simulink model "kranTest"  (R2018b)
settings: Solver=VariableStepAuto  StartTime=0.0  StopTime=Tsim  FixedStep=0.005  RelTol=1e-4
model workspace: external: MATLAB File kran_DataFile.m (data not in the file)
values from neighbouring files (symbols this model uses):
  refPointsVector = [pointThree, pointOne, pointThree, pointTwo, pointThree]    [simulate_driving.m]    (also in testDriving.m)
  Ts = 50e-3    (= 0.05)    [simulation_params.m]    (also in testDriving.m = 0.1)
undefined symbols (not defined in the file or in its folder): EvaluateTrajectory, smiData, X, Y, Z
libraries: sm_lib x105, nesl_utility x32, fl_lib x27, sh_lib x9, elec_lib x2
(part 4 of 4)

== system kranTest/Crane/Crane Mechanics/hidraulicki_trans2_2/cilindar_trans2_1_RIGID ==
  ReferenceFrame : sm_lib/Frames and Transforms/Reference Frame
  Solid : sm_lib/Body Elements/Solid  InertiaType=Custom  Mass=smiData.Solid(2).mass  MassUnits=kg  CenterOfMass=smiData.Solid(2).CoM  CenterOfMassUnits=mm  MomentsOfInertia=smiData.Solid(2).MoI  MomentsOfInertiaUnits=kg*mm^2  ProductsOfInertia=smiData.Solid(2).PoI  ProductsOfInertiaUnits=kg*mm^2  BasedOnType=Density  Density=1000  DensityUnits=kg/m^3  DoExposeReferenceFrame=on  SerializedFrames=<Frames/>  GraphicType=FromGeometry  MarkerShape=Sphere  MarkerSize=10  GraphicVisPropType=SimpleVisualProperties  GraphicDiffuseColor=smiData.Solid(2).color  GraphicSpecularColor=[0.5 0.5 0.5 1.0]  GraphicAmbientColor=[0.15 0.15 0.15 1.0]  GraphicEmissiveColor=[0.0 0.0 0.0 1.0]  GraphicShininess=75  GraphicOpacity=smiData.Solid(2).opacity  GeometryShape=FromFile  RectangleSize=[1 1]  RectangleSizeUnits=m  BrickDimensions=[1 1 1]  BrickDimensionUnits=m  CylinderRadius=1  CylinderRadiusUnits=m  CylinderLength=1  CylinderLengthUnits=m  SphereRadius=1  SphereRadiusUnits=m  EllipsoidRadii=[1 1 1]  EllipsoidRadiiUnits=m  ExtrusionCrossSection=[1 1; -1 1; -1 -1; 1 -1]  ExtrusionCrossSectionUnits=m  ExtrusionLength=1  ExtrusionLengthUnits=m  PolygonNumSides=3  PolygonOuterRadius=1  PolygonOuterRadiusUnits=m  ExtGeomFileType=STEP  ExtGeomFileName=STEPfiles/cilindar_trans2_Default_sldprt.STEP  ExtGeomFileUnits=m  RevolutionCrossSection=[1 1; 1 -1; 2 -1; 2 1]  RevolutionCrossSectionUnits=m  RevolutionExtent=Full  RevolutionAngle=180  RevolutionAngleUnits=deg
  Transform : sm_lib/Frames and Transforms/Rigid Transform  TranslationMethod=Cartesian  TranslationStandardOffset=0  TranslationLengthUnit=mm  TranslationStandardAxis=+Z  TranslationCartesianOffset=smiData.RigidTransform(2).translation  TranslationROffset=0  TranslationROffsetUnits=m  TranslationZOffset=0  TranslationZOffsetUnits=m  TranslationThetaOffset=0  TranslationThetaOffsetUnits=deg  RotationMethod=ArbitraryAxis  RotationAngleUnits=rad  RotationStandardAxis=+Z  RotationAngle=smiData.RigidTransform(2).angle  RotationArbitraryAxis=smiData.RigidTransform(2).axis  FollAlignAxisA=+X  BaseAlignAxisA=+Y  FollAlignAxisB=+Y  BaseAlignAxisB=+Z  RotationSequenceAxes=FollowerAxes  RotationSequence=XYX  RotationSequenceAngles=[0 0 0]  RotationSequenceAnglesUnits=deg  RotationMatrix=[1 0 0; 0 1 0; 0 0 1]
  Transform1 : sm_lib/Frames and Transforms/Rigid Transform  TranslationMethod=Cartesian  TranslationStandardOffset=0  TranslationLengthUnit=mm  TranslationStandardAxis=+Z  TranslationCartesianOffset=smiData.RigidTransform(20).translation  TranslationROffset=0  TranslationROffsetUnits=m  TranslationZOffset=0  TranslationZOffsetUnits=m  TranslationThetaOffset=0  TranslationThetaOffsetUnits=deg  RotationMethod=ArbitraryAxis  RotationAngleUnits=rad  RotationStandardAxis=+Z  RotationAngle=smiData.RigidTransform(20).angle  RotationArbitraryAxis=smiData.RigidTransform(20).axis  FollAlignAxisA=+X  BaseAlignAxisA=+Y  FollAlignAxisB=+Y  BaseAlignAxisB=+Z  RotationSequenceAxes=FollowerAxes  RotationSequence=XYX  RotationSequenceAngles=[0 0 0]  RotationSequenceAnglesUnits=deg  RotationMatrix=[1 0 0; 0 1 0; 0 0 1]
  F2 : PMIOPort  Side=Left
  F1 : PMIOPort  Port=2  Side=Left
  F : PMIOPort  Port=3  Side=Left
  connections:
  Solid/RConn1 -- ReferenceFrame/RConn1 -- Transform/LConn1 -- Transform1/LConn1 -- F2/RConn1
  Transform/RConn1 -- F/RConn1
  Transform1/RConn1 -- F1/RConn1

== system kranTest/Crane/Crane Mechanics/hidraulicki_trans2_2/klip_trans2_1_RIGID ==
  ReferenceFrame : sm_lib/Frames and Transforms/Reference Frame
  Solid : sm_lib/Body Elements/Solid  InertiaType=Custom  Mass=smiData.Solid(3).mass  MassUnits=kg  CenterOfMass=smiData.Solid(3).CoM  CenterOfMassUnits=mm  MomentsOfInertia=smiData.Solid(3).MoI  MomentsOfInertiaUnits=kg*mm^2  ProductsOfInertia=smiData.Solid(3).PoI  ProductsOfInertiaUnits=kg*mm^2  BasedOnType=Density  Density=1000  DensityUnits=kg/m^3  DoExposeReferenceFrame=on  SerializedFrames=<Frames/>  GraphicType=FromGeometry  MarkerShape=Sphere  MarkerSize=10  GraphicVisPropType=SimpleVisualProperties  GraphicDiffuseColor=smiData.Solid(3).color  GraphicSpecularColor=[0.5 0.5 0.5 1.0]  GraphicAmbientColor=[0.15 0.15 0.15 1.0]  GraphicEmissiveColor=[0.0 0.0 0.0 1.0]  GraphicShininess=75  GraphicOpacity=smiData.Solid(3).opacity  GeometryShape=FromFile  RectangleSize=[1 1]  RectangleSizeUnits=m  BrickDimensions=[1 1 1]  BrickDimensionUnits=m  CylinderRadius=1  CylinderRadiusUnits=m  CylinderLength=1  CylinderLengthUnits=m  SphereRadius=1  SphereRadiusUnits=m  EllipsoidRadii=[1 1 1]  EllipsoidRadiiUnits=m  ExtrusionCrossSection=[1 1; -1 1; -1 -1; 1 -1]  ExtrusionCrossSectionUnits=m  ExtrusionLength=1  ExtrusionLengthUnits=m  PolygonNumSides=3  PolygonOuterRadius=1  PolygonOuterRadiusUnits=m  ExtGeomFileType=STEP  ExtGeomFileName=STEPfiles/klip_trans2_Default_sldprt.STEP  ExtGeomFileUnits=m  RevolutionCrossSection=[1 1; 1 -1; 2 -1; 2 1]  RevolutionCrossSectionUnits=m  RevolutionExtent=Full  RevolutionAngle=180  RevolutionAngleUnits=deg
  Transform : sm_lib/Frames and Transforms/Rigid Transform  TranslationMethod=Cartesian  TranslationStandardOffset=0  TranslationLengthUnit=mm  TranslationStandardAxis=+Z  TranslationCartesianOffset=smiData.RigidTransform(1).translation  TranslationROffset=0  TranslationROffsetUnits=m  TranslationZOffset=0  TranslationZOffsetUnits=m  TranslationThetaOffset=0  TranslationThetaOffsetUnits=deg  RotationMethod=ArbitraryAxis  RotationAngleUnits=rad  RotationStandardAxis=+Z  RotationAngle=smiData.RigidTransform(1).angle  RotationArbitraryAxis=smiData.RigidTransform(1).axis  FollAlignAxisA=+X  BaseAlignAxisA=+Y  FollAlignAxisB=+Y  BaseAlignAxisB=+Z  RotationSequenceAxes=FollowerAxes  RotationSequence=XYX  RotationSequenceAngles=[0 0 0]  RotationSequenceAnglesUnits=deg  RotationMatrix=[1 0 0; 0 1 0; 0 0 1]
  Transform1 : sm_lib/Frames and Transforms/Rigid Transform  TranslationMethod=Cartesian  TranslationStandardOffset=0  TranslationLengthUnit=mm  TranslationStandardAxis=+Z  TranslationCartesianOffset=smiData.RigidTransform(10).translation  TranslationROffset=0  TranslationROffsetUnits=m  TranslationZOffset=0  TranslationZOffsetUnits=m  TranslationThetaOffset=0  TranslationThetaOffsetUnits=deg  RotationMethod=ArbitraryAxis  RotationAngleUnits=rad  RotationStandardAxis=+Z  RotationAngle=smiData.RigidTransform(10).angle  RotationArbitraryAxis=smiData.RigidTransform(10).axis  FollAlignAxisA=+X  BaseAlignAxisA=+Y  FollAlignAxisB=+Y  BaseAlignAxisB=+Z  RotationSequenceAxes=FollowerAxes  RotationSequence=XYX  RotationSequenceAngles=[0 0 0]  RotationSequenceAnglesUnits=deg  RotationMatrix=[1 0 0; 0 1 0; 0 0 1]
  F1 : PMIOPort  Side=Left
  F : PMIOPort  Port=2  Side=Right
  connections:
  Solid/RConn1 -- ReferenceFrame/RConn1 -- Transform/LConn1 -- Transform1/LConn1
  Transform/RConn1 -- F/RConn1
  Transform1/RConn1 -- F1/RConn1

== matlab function kranTest/ControllerTrans1/RegulatorTrans1 ==
  data: t input; coordNum input; y output; pos input; vel input; load_pos input; load_vel input; top_pos input; top_vel input
function y = trans1(t, coordNum, pos, vel, load_pos, load_vel, top_pos, top_vel)

% Hardcode references
actuatorRefOne = [0, 0.7, 3.4, 3.4, 6150];
actuatorRefTwo = [-135, 0.415, 3.4, 3.4, 4300];
actuatorRefThree = [-90, 0.8, 0, 0, 2000];
actuatorRefVector = [actuatorRefThree; actuatorRefOne,; actuatorRefThree; actuatorRefTwo; actuatorRefThree];

baseRef = actuatorRefVector(coordNum, 1);
rotRef = actuatorRefVector(coordNum, 2);
trans1Ref = actuatorRefVector(coordNum, 3);
trans2Ref = actuatorRefVector(coordNum, 4);
pulleyRef = actuatorRefVector(coordNum, 5);

% Measurement extraction
rotPos = pos(1);
trans1Pos = pos(2);
trans2Pos = pos(3);
baseAngle = pos(4);
pulleyAngle = pos(5);

rotVel = vel(1);
tran1Vel = vel(2);
trans2Vel = vel(3);
baseVel = vel(4);
pulleyVel = vel(5);

deltaRot = rotRef - rotPos;
if (abs(deltaRot) > 0.005)
    y = 0;
else
    deltaTrans1 = trans1Ref - trans1Pos;
    if(abs(deltaTrans1) <= 0.005)
        y = 0;
    else
        y = 0.005*sign(deltaTrans1);
    end
end

end

== matlab function kranTest/ControllerRot/RegulatorRot ==
  data: t input; coordNum input; y output; pos input; vel input; load_pos input; load_vel input; top_pos input; top_vel input
function y = rot(t, coordNum, pos, vel, load_pos, load_vel, top_pos, top_vel)

% Hardcode references
actuatorRefOne = [0, 0.7, 3.4, 3.4, 6150];
actuatorRefTwo = [-135, 0.415, 3.4, 3.4, 4300];
actuatorRefThree = [-90, 0.8, 0, 0, 2000];
actuatorRefVector = [actuatorRefThree; actuatorRefOne,; actuatorRefThree; actuatorRefTwo; actuatorRefThree];

baseRef = actuatorRefVector(coordNum, 1);
rotRef = actuatorRefVector(coordNum, 2);
trans1Ref = actuatorRefVector(coordNum, 3);
trans2Ref = actuatorRefVector(coordNum, 4);
pulleyRef = actuatorRefVector(coordNum, 5);

% Measurement extraction
rotPos = pos(1);
trans1Pos = pos(2);
trans2Pos = pos(3);
baseAngle = pos(4);
pulleyAngle = pos(5);

rotVel = vel(1);
tran1Vel = vel(2);
trans2Vel = vel(3);
baseVel = vel(4);
pulleyVel = vel(5);

delta = rotRef - rotPos;
if(abs(delta) <= 0.005)
    y = 0;
else
    y = 0.003*sign(delta);
end

end

== matlab function kranTest/ControllerTrans2/RegulatorTrans2 ==
  data: t input; coordNum input; y output; pos input; vel input; load_pos input; load_vel input; top_pos input; top_vel input
function y = trans2(t, coordNum, pos, vel, load_pos, load_vel, top_pos, top_vel)

% Hardcode references
actuatorRefOne = [0, 0.7, 3.4, 3.4, 6150];
actuatorRefTwo = [-135, 0.415, 3.4, 3.4, 4300];
actuatorRefThree = [-90, 0.8, 0, 0, 2000];
actuatorRefVector = [actuatorRefThree; actuatorRefOne,; actuatorRefThree; actuatorRefTwo; actuatorRefThree];

baseRef = actuatorRefVector(coordNum, 1);
rotRef = actuatorRefVector(coordNum, 2);
trans1Ref = actuatorRefVector(coordNum, 3);
trans2Ref = actuatorRefVector(coordNum, 4);
pulleyRef = actuatorRefVector(coordNum, 5);

% Measurement extraction
rotPos = pos(1);
trans1Pos = pos(2);
trans2Pos = pos(3);
baseAngle = pos(4);
pulleyAngle = pos(5);

rotVel = vel(1);
tran1Vel = vel(2);
trans2Vel = vel(3);
baseVel = vel(4);
pulleyVel = vel(5);

deltaRot = rotRef - rotPos;
deltaTrans1 = trans1Ref - trans1Pos;
if (abs(deltaRot) > 0.005 || abs(deltaTrans1) > 0.005)
    y = 0;
else
    deltaTrans2 = trans2Ref - trans2Pos;
    if(abs(deltaTrans2) <= 0.005)
        y = 0;
    else
        y = 0.005*sign(deltaTrans2);
    end
end

end

== matlab function kranTest/ControllerBase/RegulatorBase ==
  data: t input; coordNum input; y output; pos input; vel input; load_pos input; load_vel input; top_pos input; top_vel input
function y = base(t, coordNum, pos, vel, load_pos, load_vel, top_pos, top_vel)

% Hardcode references
actuatorRefOne = [0, 0.7, 3.4, 3.4, 6150];
actuatorRefTwo = [-135, 0.415, 3.4, 3.4, 4300];
actuatorRefThree = [-90, 0.8, 0, 0, 2000];
actuatorRefVector = [actuatorRefThree; actuatorRefOne,; actuatorRefThree; actuatorRefTwo; actuatorRefThree];

baseRef = actuatorRefVector(coordNum, 1);
rotRef = actuatorRefVector(coordNum, 2);
trans1Ref = actuatorRefVector(coordNum, 3);
trans2Ref = actuatorRefVector(coordNum, 4);
pulleyRef = actuatorRefVector(coordNum, 5);

% Measurement extraction
rotPos = pos(1);
trans1Pos = pos(2);
trans2Pos = pos(3);
baseAngle = pos(4);
pulleyAngle = pos(5);

rotVel = vel(1);
tran1Vel = vel(2);
trans2Vel = vel(3);
baseVel = vel(4);
pulleyVel = vel(5);

deltaTrans2 = trans2Ref - trans2Pos;
delta = baseRef/180*pi - baseAngle;
y = 150*delta;

end

== matlab function kranTest/ControllerPulley/RegulatorPulley ==
  data: t input; coordNum input; y output; pos input; vel input; load_pos input; load_vel input; top_pos input; top_vel input
function y = pulley(t, coordNum, pos, vel, load_pos, load_vel, top_pos, top_vel)

% Hardcode references
actuatorRefOne = [0, 0.7, 3.4, 3.4, 6150];
actuatorRefTwo = [-135, 0.415, 3.4, 3.4, 4300];
actuatorRefThree = [-90, 0.8, 0, 0, 2000];
actuatorRefVector = [actuatorRefThree; actuatorRefOne,; actuatorRefThree; actuatorRefTwo; actuatorRefThree];

baseRef = actuatorRefVector(coordNum, 1);
rotRef = actuatorRefVector(coordNum, 2);
trans1Ref = actuatorRefVector(coordNum, 3);
trans2Ref = actuatorRefVector(coordNum, 4);
pulleyRef = actuatorRefVector(coordNum, 5);

% Measurement extraction
rotPos = pos(1);
trans1Pos = pos(2);
trans2Pos = pos(3);
baseAngle = pos(4);
pulleyAngle = pos(5);

rotVel = vel(1);
tran1Vel = vel(2);
trans2Vel = vel(3);
baseVel = vel(4);
pulleyVel = vel(5);

%newRef = pulleyRef + (trans1Ref + trans2Ref)/(0.135*pi)*180;

deltaTrans1 = trans1Ref - trans1Pos;
if(abs(deltaTrans1) > 0.05)
    pulleyRef = pulleyRef + 2000;
end
    
delta = pulleyRef/180*pi - pulleyAngle;
y = -100*delta;
    
end
